simulink model "Scratch3"  (Simulink 8.5)
settings: Solver=ode4  StartTime=0.0  StopTime=20  FixedStep=0.005  RelTol=1e-3
libraries: dspinverses x1, roblocks x1
(part 2 of 3)

== matlab function Christoffle Matrix (C) ==
  data: q1d input double; q2d input double; q3d input double; q4d input double; q1 input double; C_Num output double; q2 input double; q3 input double; q4 input double; q1dd input double; q2dd input double; q3dd input double; q4dd input double; Cdot_Num output double
function [C_Num,Cdot_Num] = fcn(q1d, q2d, q3d, q4d, q1, q2, q3, q4, q1dd, q2dd, q3dd, q4dd)
%#codegen
% coder.extrinsic('evalin');
% coder.extrinsic('subs'); 
% coder.extrinsic('eval'); 
% 
% StatesSym1 = evalin('base','states1');
% StatesSym2 = evalin('base','states2');
% 
% Csym = evalin('base','C');
% Cdotsym = evalin('base','Cdot');
% 
% 
% States_Num1 = [q1t;q2t;q3t;q4t;q1dt;q2dt;q3dt;q4dt];
% States_Num2 = [q1t;q2t;q3t;q4t;q1dt;q2dt;q3dt;q4dt;q1ddt;q2ddt;q3ddt;q4ddt];
% 
% C_Num = zeros(4,1);
% Cdot_Num = zeros(4,1);
% C_Num = eval(subs(Csym,StatesSym1,States_Num1));
% Cdot_Num = eval(subs(Cdotsym,StatesSym2,States_Num2));

m2 = 7;
m3 = 7;
m4 = 5;
l1 = 1;
l2 = 0.7;
l3 = 0.7; 
l4 = 0.5;
d2 = l2/2;
d3 = l3/2; 
d4 = l4/2;


C_Num = [- q4d*(q1d*(d4*l2*m4*sin(q3 + q4) + d4*l3*m4*sin(q4) + d4*l1*m4*sin(q2 + q3 + q4)) + q2d*(d4*l2*m4*sin(q3 + q4) + d4*l3*m4*sin(q4) + d4*l1*m4*sin(q2 + q3 + q4)) + q3d*(d4*l2*m4*sin(q3 + q4) + d4*l3*m4*sin(q4) + d4*l1*m4*sin(q2 + q3 + q4)) + q4d*(d4*l2*m4*sin(q3 + q4) + d4*l3*m4*sin(q4) + d4*l1*m4*sin(q2 + q3 + q4))) - q2d*(q2d*(d3*l1*m3*sin(q2 + q3) - (l1^2*m2*sin(2*q1))/2 - (d2^2*m2*sin(2*q1 + 2*q2))/2 + l1*l3*m4*sin(q2 + q3) + (d2*l1*m2*sin(q2))/2 + l1*l2*m3*sin(q2) + l1*l2*m4*sin(q2) - (d2*l1*m2*sin(2*q1 + q2))/2 + d4*l1*m4*sin(q2 + q3 + q4)) + q4d*(d4*l2*m4*sin(q3 + q4) + d4*l3*m4*sin(q4) + d4*l1*m4*sin(q2 + q3 + q4)) + q1d*(d3*l1*m3*sin(q2 + q3) - (d2^2*m2*sin(2*q1 + 2*q2))/2 + l1*l3*m4*sin(q2 + q3) + (d2*l1*m2*sin(q2))/2 + l1*l2*m3*sin(q2) + l1*l2*m4*sin(q2) - (d2*l1*m2*sin(2*q1 + q2))/2 + d4*l1*m4*sin(q2 + q3 + q4)) + q3d*(d3*l1*m3*sin(q2 + q3) + d4*l2*m4*sin(q3 + q4) + l1*l3*m4*sin(q2 + q3) + d3*l2*m3*sin(q3) + l2*l3*m4*sin(q3) + d4*l1*m4*sin(q2 + q3 + q4))) - q1d*(q4d*(d4*l2*m4*sin(q3 + q4) + d4*l3*m4*sin(q4) + d4*l1*m4*sin(q2 + q3 + q4)) - q1d*((m2*sin(2*q1 + 2*q2)*d2^2)/2 + m2*sin(2*q1 + q2)*d2*l1 + (m2*sin(2*q1)*l1^2)/2) + q2d*(d3*l1*m3*sin(q2 + q3) - (d2^2*m2*sin(2*q1 + 2*q2))/2 + l1*l3*m4*sin(q2 + q3) + (d2*l1*m2*sin(q2))/2 + l1*l2*m3*sin(q2) + l1*l2*m4*sin(q2) - (d2*l1*m2*sin(2*q1 + q2))/2 + d4*l1*m4*sin(q2 + q3 + q4)) + q3d*(d3*l1*m3*sin(q2 + q3) + d4*l2*m4*sin(q3 + q4) + l1*l3*m4*sin(q2 + q3) + d3*l2*m3*sin(q3) + l2*l3*m4*sin(q3) + d4*l1*m4*sin(q2 + q3 + q4))) - q3d*(q4d*(d4*l2*m4*sin(q3 + q4) + d4*l3*m4*sin(q4) + d4*l1*m4*sin(q2 + q3 + q4)) + q1d*(d3*l1*m3*sin(q2 + q3) + d4*l2*m4*sin(q3 + q4) + l1*l3*m4*sin(q2 + q3) + d3*l2*m3*sin(q3) + l2*l3*m4*sin(q3) + d4*l1*m4*sin(q2 + q3 + q4)) + q2d*(d3*l1*m3*sin(q2 + q3) + d4*l2*m4*sin(q3 + q4) + l1*l3*m4*sin(q2 + q3) + d3*l2*m3*sin(q3) + l2*l3*m4*sin(q3) + d4*l1*m4*sin(q2 + q3 + q4)) + q3d*(d3*l1*m3*sin(q2 + q3) + d4*l2*m4*sin(q3 + q4) + l1*l3*m4*sin(q2 + q3) + d3*l2*m3*sin(q3) + l2*l3*m4*sin(q3) + d4*l1*m4*sin(q2 + q3 + q4)))
                                                                                                                                                                                                                                                                                                                                                                                                                                                                                                                                                                                                                                                                                                                                                                                                                                                                                                                                                                                         - q4d*(q1d*(d4*l2*m4*sin(q3 + q4) + d4*l3*m4*sin(q4)) + q2d*(d4*l2*m4*sin(q3 + q4) + d4*l3*m4*sin(q4)) + q3d*(d4*l2*m4*sin(q3 + q4) + d4*l3*m4*sin(q4)) + q4d*(d4*l2*m4*sin(q3 + q4) + d4*l3*m4*sin(q4))) - q2d*(q4d*(d4*l2*m4*sin(q3 + q4) + d4*l3*m4*sin(q4)) - q1d*((m2*sin(2*q1 + 2*q2)*d2^2)/2 - (l1^2*m2*sin(2*q1))/2) + q3d*(d4*l2*m4*sin(q3 + q4) + d3*l2*m3*sin(q3) + l2*l3*m4*sin(q3)) - (d2^2*m2*q2d*sin(2*q1 + 2*q2))/2) - q1d*(q4d*(d4*l2*m4*sin(q3 + q4) + d4*l3*m4*sin(q4)) - q2d*((m2*sin(2*q1 + 2*q2)*d2^2)/2 - (l1^2*m2*sin(2*q1))/2) + q3d*(d4*l2*m4*sin(q3 + q4) + d3*l2*m3*sin(q3) + l2*l3*m4*sin(q3)) - q1d*((d2^2*m2*sin(2*q1 + 2*q2))/2 + d3*l1*m3*sin(q2 + q3) + l1*l3*m4*sin(q2 + q3) + (d2*l1*m2*sin(q2))/2 + l1*l2*m3*sin(q2) + l1*l2*m4*sin(q2) + (d2*l1*m2*sin(2*q1 + q2))/2 + d4*l1*m4*sin(q2 + q3 + q4))) - q3d*(q4d*(d4*l2*m4*sin(q3 + q4) + d4*l3*m4*sin(q4)) + q1d*(d4*l2*m4*sin(q3 + q4) + d3*l2*m3*sin(q3) + l2*l3*m4*sin(q3)) + q2d*(d4*l2*m4*sin(q3 + q4) + d3*l2*m3*sin(q3) + l2*l3*m4*sin(q3)) + q3d*(d4*l2*m4*sin(q3 + q4) + d3*l2*m3*sin(q3) + l2*l3*m4*sin(q3)))
                                                                                                                                                                                                                                                                                                                                                                                                                                                                                                                                                                                                                                                                                                                                                                                                                                                                                                                                                                                                                                                                                                                                                                                                                                                                                                                                                                                                                                                                                                                                                    q2d*(q1d*(d4*l2*m4*sin(q3 + q4) + d3*l2*m3*sin(q3) + l2*l3*m4*sin(q3)) + q2d*(d4*l2*m4*sin(q3 + q4) + d3*l2*m3*sin(q3) + l2*l3*m4*sin(q3)) - d4*l3*m4*q4d*sin(q4)) + q1d*(q2d*(d4*l2*m4*sin(q3 + q4) + d3*l2*m3*sin(q3) + l2*l3*m4*sin(q3)) + q1d*(d3*l1*m3*sin(q2 + q3) + d4*l2*m4*sin(q3 + q4) + l1*l3*m4*sin(q2 + q3) + d3*l2*m3*sin(q3) + l2*l3*m4*sin(q3) + d4*l1*m4*sin(q2 + q3 + q4)) - d4*l3*m4*q4d*sin(q4)) - q4d*(d4*l3*m4*q1d*sin(q4) + d4*l3*m4*q2d*sin(q4) + d4*l3*m4*q3d*sin(q4) + d4*l3*m4*q4d*sin(q4)) - d4*l3*m4*q3d*q4d*sin(q4)
                                                                                                                                                                                                                                                                                                                                                                                                                                                                                                                                                                                                                                                                                                                                                                                                                                                                                                                                                                                                                                                                                                                                                                                                                                                                                                                                                                                                                                                                                                                                                    q2d*(q1d*(d4*l2*m4*sin(q3 + q4) + d3*l2*m3*sin(q3) + l2*l3*m4*sin(q3)) + q2d*(d4*l2*m4*sin(q3 + q4) + d3*l2*m3*sin(q3) + l2*l3*m4*sin(q3)) - d4*l3*m4*q4d*sin(q4)) + q1d*(q2d*(d4*l2*m4*sin(q3 + q4) + d3*l2*m3*sin(q3) + l2*l3*m4*sin(q3)) + q1d*(d3*l1*m3*sin(q2 + q3) + d4*l2*m4*sin(q3 + q4) + l1*l3*m4*sin(q2 + q3) + d3*l2*m3*sin(q3) + l2*l3*m4*sin(q3) + d4*l1*m4*sin(q2 + q3 + q4)) - d4*l3*m4*q4d*sin(q4)) - q4d*(d4*l3*m4*q1d*sin(q4) + d4*l3*m4*q2d*sin(q4) + d4*l3*m4*q3d*sin(q4) + d4*l3*m4*q4d*sin(q4)) - d4*l3*m4*q3d*q4d*sin(q4)];

Cdot_Num = [q1d*(q2d*(q2d*(m2*cos(2*q1 + 2*q2)*d2^2 + m2*cos(2*q1 + q2)*d2*l1 + m2*cos(2*q1)*l1^2) + q1d*(m2*cos(2*q1 + 2*q2)*d2^2 + l1*m2*cos(2*q1 + q2)*d2)) + q1d*(q1d*(m2*cos(2*q1 + 2*q2)*d2^2 + 2*m2*cos(2*q1 + q2)*d2*l1 + m2*cos(2*q1)*l1^2) + q2d*(m2*cos(2*q1 + 2*q2)*d2^2 + l1*m2*cos(2*q1 + q2)*d2))) - q3d*(q3d*(q4d*(d4*l2*m4*cos(q3 + q4) + d4*l1*m4*cos(q2 + q3 + q4)) + q1d*(d3*l1*m3*cos(q2 + q3) + d4*l2*m4*cos(q3 + q4) + l1*l3*m4*cos(q2 + q3) + d3*l2*m3*cos(q3) + l2*l3*m4*cos(q3) + d4*l1*m4*cos(q2 + q3 + q4)) + q2d*(d3*l1*m3*cos(q2 + q3) + d4*l2*m4*cos(q3 + q4) + l1*l3*m4*cos(q2 + q3) + d3*l2*m3*cos(q3) + l2*l3*m4*cos(q3) + d4*l1*m4*cos(q2 + q3 + q4)) + q3d*(d3*l1*m3*cos(q2 + q3) + d4*l2*m4*cos(q3 + q4) + l1*l3*m4*cos(q2 + q3) + d3*l2*m3*cos(q3) + l2*l3*m4*cos(q3) + d4*l1*m4*cos(q2 + q3 + q4))) + q1d*(q4d*(d4*l2*m4*cos(q3 + q4) + d4*l1*m4*cos(q2 + q3 + q4)) + q2d*(d3*l1*m3*cos(q2 + q3) + l1*l3*m4*cos(q2 + q3) + d4*l1*m4*cos(q2 + q3 + q4)) + q3d*(d3*l1*m3*cos(q2 + q3) + d4*l2*m4*cos(q3 + q4) + l1*l3*m4*cos(q2 + q3) + d3*l2*m3*cos(q3) + l2*l3*m4*cos(q3) + d4*l1*m4*cos(q2 + q3 + q4))) + q4d*(q1d*(d4*l2*m4*cos(q3 + q4) + d4*l1*m4*cos(q2 + q3 + q4)) + q2d*(d4*l2*m4*cos(q3 + q4) + d4*l1*m4*cos(q2 + q3 + q4)) + q3d*(d4*l2*m4*cos(q3 + q4) + d4*l1*m4*cos(q2 + q3 + q4)) + q4d*(d4*l2*m4*cos(q3 + q4) + d4*l1*m4*cos(q2 + q3 + q4))) + q2d*(q4d*(d4*l2*m4*cos(q3 + q4) + d4*l1*m4*cos(q2 + q3 + q4)) + q1d*(d3*l1*m3*cos(q2 + q3) + l1*l3*m4*cos(q2 + q3) + d4*l1*m4*cos(q2 + q3 + q4)) + q2d*(d3*l1*m3*cos(q2 + q3) + l1*l3*m4*cos(q2 + q3) + d4*l1*m4*cos(q2 + q3 + q4)) + q3d*(d3*l1*m3*cos(q2 + q3) + d4*l2*m4*cos(q3 + q4) + l1*l3*m4*cos(q2 + q3) + d3*l2*m3*cos(q3) + l2*l3*m4*cos(q3) + d4*l1*m4*cos(q2 + q3 + q4)))) - q4d*(q1d*(q3d*(d4*l2*m4*cos(q3 + q4) + d4*l1*m4*cos(q2 + q3 + q4)) + q4d*(d4*l2*m4*cos(q3 + q4) + d4*l3*m4*cos(q4) + d4*l1*m4*cos(q2 + q3 + q4)) + d4*l1*m4*q2d*cos(q2 + q3 + q4)) + q2d*(q3d*(d4*l2*m4*cos(q3 + q4) + d4*l1*m4*cos(q2 + q3 + q4)) + q4d*(d4*l2*m4*cos(q3 + q4) + d4*l3*m4*cos(q4) + d4*l1*m4*cos(q2 + q3 + q4)) + d4*l1*m4*q1d*cos(q2 + q3 + q4) + d4*l1*m4*q2d*cos(q2 + q3 + q4)) + q3d*(q1d*(d4*l2*m4*cos(q3 + q4) + d4*l1*m4*cos(q2 + q3 + q4)) + q2d*(d4*l2*m4*cos(q3 + q4) + d4*l1*m4*cos(q2 + q3 + q4)) + q3d*(d4*l2*m4*cos(q3 + q4) + d4*l1*m4*cos(q2 + q3 + q4)) + q4d*(d4*l2*m4*cos(q3 + q4) + d4*l3*m4*cos(q4) + d4*l1*m4*cos(q2 + q3 + q4))) + q4d*(q1d*(d4*l2*m4*cos(q3 + q4) + d4*l3*m4*cos(q4) + d4*l1*m4*cos(q2 + q3 + q4)) + q2d*(d4*l2*m4*cos(q3 + q4) + d4*l3*m4*cos(q4) + d4*l1*m4*cos(q2 + q3 + q4)) + q3d*(d4*l2*m4*cos(q3 + q4) + d4*l3*m4*cos(q4) + d4*l1*m4*cos(q2 + q3 + q4)) + q4d*(d4*l2*m4*cos(q3 + q4) + d4*l3*m4*cos(q4) + d4*l1*m4*cos(q2 + q3 + q4)))) - q4dd*(2*q1d*(d4*l2*m4*sin(q3 + q4) + d4*l3*m4*sin(q4) + d4*l1*m4*sin(q2 + q3 + q4)) + 2*q2d*(d4*l2*m4*sin(q3 + q4) + d4*l3*m4*sin(q4) + d4*l1*m4*sin(q2 + q3 + q4)) + 2*q3d*(d4*l2*m4*sin(q3 + q4) + d4*l3*m4*sin(q4) + d4*l1*m4*sin(q2 + q3 + q4)) + 2*q4d*(d4*l2*m4*sin(q3 + q4) + d4*l3*m4*sin(q4) + d4*l1*m4*sin(q2 + q3 + q4))) - q2dd*(2*q2d*(d3*l1*m3*sin(q2 + q3) - (l1^2*m2*sin(2*q1))/2 - (d2^2*m2*sin(2*q1 + 2*q2))/2 + l1*l3*m4*sin(q2 + q3) + (d2*l1*m2*sin(q2))/2 + l1*l2*m3*sin(q2) + l1*l2*m4*sin(q2) - (d2*l1*m2*sin(2*q1 + q2))/2 + d4*l1*m4*sin(q2 + q3 + q4)) + 2*q4d*(d4*l2*m4*sin(q3 + q4) + d4*l3*m4*sin(q4) + d4*l1*m4*sin(q2 + q3 + q4)) + 2*q1d*(d3*l1*m3*sin(q2 + q3) - (d2^2*m2*sin(2*q1 + 2*q2))/2 + l1*l3*m4*sin(q2 + q3) + (d2*l1*m2*sin(q2))/2 + l1*l2*m3*sin(q2) + l1*l2*m4*sin(q2) - (d2*l1*m2*sin(2*q1 + q2))/2 + d4*l1*m4*sin(q2 + q3 + q4)) + 2*q3d*(d3*l1*m3*sin(q2 + q3) + d4*l2*m4*sin(q3 + q4) + l1*l3*m4*sin(q2 + q3) + d3*l2*m3*sin(q3) + l2*l3*m4*sin(q3) + d4*l1*m4*sin(q2 + q3 + q4))) - q1dd*(2*q4d*(d4*l2*m4*sin(q3 + q4) + d4*l3*m4*sin(q4) + d4*l1*m4*sin(q2 + q3 + q4)) - 2*q1d*((m2*sin(2*q1 + 2*q2)*d2^2)/2 + m2*sin(2*q1 + q2)*d2*l1 + (m2*sin(2*q1)*l1^2)/2) + 2*q2d*(d3*l1*m3*sin(q2 + q3) - (d2^2*m2*sin(2*q1 + 2*q2))/2 + l1*l3*m4*sin(q2 + q3) + (d2*l1*m2*sin(q2))/2 + l1*l2*m3*sin(q2) + l1*l2*m4*sin(q2) - (d2*l1*m2*sin(2*q1 + q2))/2 + d4*l1*m4*sin(q2 + q3 + q4)) + 2*q3d*(d3*l1*m3*sin(q2 + q3) + d4*l2*m4*sin(q3 + q4) + l1*l3*m4*sin(q2 + q3) + d3*l2*m3*sin(q3) + l2*l3*m4*sin(q3) + d4*l1*m4*sin(q2 + q3 + q4))) - q3dd*(2*q4d*(d4*l2*m4*sin(q3 + q4) + d4*l3*m4*sin(q4) + d4*l1*m4*sin(q2 + q3 + q4)) + 2*q1d*(d3*l1*m3*sin(q2 + q3) + d4*l2*m4*sin(q3 + q4) + l1*l3*m4*sin(q2 + q3) + d3*l2*m3*sin(q3) + l2*l3*m4*sin(q3) + d4*l1*m4*sin(q2 + q3 + q4)) + 2*q2d*(d3*l1*m3*sin(q2 + q3) + d4*l2*m4*sin(q3 + q4) + l1*l3*m4*sin(q2 + q3) + d3*l2*m3*sin(q3) + l2*l3*m4*sin(q3) + d4*l1*m4*sin(q2 + q3 + q4)) + 2*q3d*(d3*l1*m3*sin(q2 + q3) + d4*l2*m4*sin(q3 + q4) + l1*l3*m4*sin(q2 + q3) + d3*l2*m3*sin(q3) + l2*l3*m4*sin(q3) + d4*l1*m4*sin(q2 + q3 + q4))) - q2d*(q2d*(q1d*(d3*l1*m3*cos(q2 + q3) - d2^2*m2*cos(2*q1 + 2*q2) + l1*l3*m4*cos(q2 + q3) + (d2*l1*m2*cos(q2))/2 + l1*l2*m3*cos(q2) + l1*l2*m4*cos(q2) - (d2*l1*m2*cos(2*q1 + q2))/2 + d4*l1*m4*cos(q2 + q3 + q4)) + q2d*(d3*l1*m3*cos(q2 + q3) - d2^2*m2*cos(2*q1 + 2*q2) + l1*l3*m4*cos(q2 + q3) + (d2*l1*m2*cos(q2))/2 + l1*l2*m3*cos(q2) + l1*l2*m4*cos(q2) - (d2*l1*m2*cos(2*q1 + q2))/2 + d4*l1*m4*cos(q2 + q3 + q4)) + q3d*(d3*l1*m3*cos(q2 + q3) + l1*l3*m4*cos(q2 + q3) + d4*l1*m4*cos(q2 + q3 + q4)) + d4*l1*m4*q4d*cos(q2 + q3 + q4)) + q3d*(q1d*(d3*l1*m3*cos(q2 + q3) + l1*l3*m4*cos(q2 + q3) + d4*l1*m4*cos(q2 + q3 + q4)) + q2d*(d3*l1*m3*cos(q2 + q3) + l1*l3*m4*cos(q2 + q3) + d4*l1*m4*cos(q2 + q3 + q4)) + q3d*(d3*l1*m3*cos(q2 + q3) + l1*l3*m4*cos(q2 + q3) + d4*l1*m4*cos(q2 + q3 + q4)) + d4*l1*m4*q4d*cos(q2 + q3 + q4)) + q4d*(d4*l1*m4*q1d*cos(q2 + q3 + q4) + d4*l1*m4*q2d*cos(q2 + q3 + q4) + d4*l1*m4*q3d*cos(q2 + q3 + q4) + d4*l1*m4*q4d*cos(q2 + q3 + q4)) + q1d*(q2d*(d3*l1*m3*cos(q2 + q3) - d2^2*m2*cos(2*q1 + 2*q2) + l1*l3*m4*cos(q2 + q3) + (d2*l1*m2*cos(q2))/2 + l1*l2*m3*cos(q2) + l1*l2*m4*cos(q2) - (d2*l1*m2*cos(2*q1 + q2))/2 + d4*l1*m4*cos(q2 + q3 + q4)) + q3d*(d3*l1*m3*cos(q2 + q3) + l1*l3*m4*cos(q2 + q3) + d4*l1*m4*cos(q2 + q3 + q4)) - q1d*(m2*cos(2*q1 + 2*q2)*d2^2 + l1*m2*cos(2*q1 + q2)*d2) + d4*l1*m4*q4d*cos(q2 + q3 + q4)))
                                                                                                                                                                                                                                                                                                                                                                                                                                                                                                                                                                                                                                                                                                                                                                                                                                                                                                                                                                                                                                                                                                                                                                                                                                                                                                                                                                                                                                                                                                                                                                                                                                                                                                                                                                                                                                                                                                                                                                                                                                                                                                                                                                                                                                                                                                                                                                                                                                                                                                                                                                                                                                                                                                                                                                                                                                                                                                                                                                                                                                                                                                                                                                                                                                                                                                                                                                                           q2d*(q1d*(q1d*(d2^2*m2*cos(2*q1 + 2*q2) + d3*l1*m3*cos(q2 + q3) + l1*l3*m4*cos(q2 + q3) + (d2*l1*m2*cos(q2))/2 + l1*l2*m3*cos(q2) + l1*l2*m4*cos(q2) + (d2*l1*m2*cos(2*q1 + q2))/2 + d4*l1*m4*cos(q2 + q3 + q4)) + d2^2*m2*q2d*cos(2*q1 + 2*q2)) + q2d*(d2^2*m2*q1d*cos(2*q1 + 2*q2) + d2^2*m2*q2d*cos(2*q1 + 2*q2))) - q3d*(q2d*(q3d*(d4*l2*m4*cos(q3 + q4) + d3*l2*m3*cos(q3) + l2*l3*m4*cos(q3)) + d4*l2*m4*q4d*cos(q3 + q4)) + q1d*(q3d*(d4*l2*m4*cos(q3 + q4) + d3*l2*m3*cos(q3) + l2*l3*m4*cos(q3)) - q1d*(d3*l1*m3*cos(q2 + q3) + l1*l3*m4*cos(q2 + q3) + d4*l1*m4*cos(q2 + q3 + q4)) + d4*l2*m4*q4d*cos(q3 + q4)) + q3d*(q1d*(d4*l2*m4*cos(q3 + q4) + d3*l2*m3*cos(q3) + l2*l3*m4*cos(q3)) + q2d*(d4*l2*m4*cos(q3 + q4) + d3*l2*m3*cos(q3) + l2*l3*m4*cos(q3)) + q3d*(d4*l2*m4*cos(q3 + q4) + d3*l2*m3*cos(q3) + l2*l3*m4*cos(q3)) + d4*l2*m4*q4d*cos(q3 + q4)) + q4d*(d4*l2*m4*q1d*cos(q3 + q4) + d4*l2*m4*q2d*cos(q3 + q4) + d4*l2*m4*q3d*cos(q3 + q4) + d4*l2*m4*q4d*cos(q3 + q4))) - q4dd*(2*q1d*(d4*l2*m4*sin(q3 + q4) + d4*l3*m4*sin(q4)) + 2*q2d*(d4*l2*m4*sin(q3 + q4) + d4*l3*m4*sin(q4)) + 2*q3d*(d4*l2*m4*sin(q3 + q4) + d4*l3*m4*sin(q4)) + 2*q4d*(d4*l2*m4*sin(q3 + q4) + d4*l3*m4*sin(q4))) - q2dd*(2*q4d*(d4*l2*m4*sin(q3 + q4) + d4*l3*m4*sin(q4)) - 2*q1d*((m2*sin(2*q1 + 2*q2)*d2^2)/2 - (l1^2*m2*sin(2*q1))/2) + 2*q3d*(d4*l2*m4*sin(q3 + q4) + d3*l2*m3*sin(q3) + l2*l3*m4*sin(q3)) - d2^2*m2*q2d*sin(2*q1 + 2*q2)) - q1d*(q2d*(q1d*(m2*cos(2*q1)*l1^2 - m2*cos(2*q1 + 2*q2)*d2^2) - d2^2*m2*q2d*cos(2*q1 + 2*q2)) - q1d*(q1d*(m2*cos(2*q1 + 2*q2)*d2^2 + l1*m2*cos(2*q1 + q2)*d2) - q2d*(m2*cos(2*q1)*l1^2 - m2*cos(2*q1 + 2*q2)*d2^2))) - q1dd*(2*q4d*(d4*l2*m4*sin(q3 + q4) + d4*l3*m4*sin(q4)) - 2*q2d*((m2*sin(2*q1 + 2*q2)*d2^2)/2 - (l1^2*m2*sin(2*q1))/2) + 2*q3d*(d4*l2*m4*sin(q3 + q4) + d3*l2*m3*sin(q3) + l2*l3*m4*sin(q3)) - 2*q1d*((d2^2*m2*sin(2*q1 + 2*q2))/2 + d3*l1*m3*sin(q2 + q3) + l1*l3*m4*sin(q2 + q3) + (d2*l1*m2*sin(q2))/2 + l1*l2*m3*sin(q2) + l1*l2*m4*sin(q2) + (d2*l1*m2*sin(2*q1 + q2))/2 + d4*l1*m4*sin(q2 + q3 + q4))) - q4d*(q3d*(q4d*(d4*l2*m4*cos(q3 + q4) + d4*l3*m4*cos(q4)) + d4*l2*m4*q1d*cos(q3 + q4) + d4*l2*m4*q2d*cos(q3 + q4) + d4*l2*m4*q3d*cos(q3 + q4)) + q4d*(q1d*(d4*l2*m4*cos(q3 + q4) + d4*l3*m4*cos(q4)) + q2d*(d4*l2*m4*cos(q3 + q4) + d4*l3*m4*cos(q4)) + q3d*(d4*l2*m4*cos(q3 + q4) + d4*l3*m4*cos(q4)) + q4d*(d4*l2*m4*cos(q3 + q4) + d4*l3*m4*cos(q4))) + q2d*(q4d*(d4*l2*m4*cos(q3 + q4) + d4*l3*m4*cos(q4)) + d4*l2*m4*q3d*cos(q3 + q4)) + q1d*(q4d*(d4*l2*m4*cos(q3 + q4) + d4*l3*m4*cos(q4)) - d4*l1*m4*q1d*cos(q2 + q3 + q4) + d4*l2*m4*q3d*cos(q3 + q4))) - q3dd*(2*q4d*(d4*l2*m4*sin(q3 + q4) + d4*l3*m4*sin(q4)) + 2*q1d*(d4*l2*m4*sin(q3 + q4) + d3*l2*m3*sin(q3) + l2*l3*m4*sin(q3)) + 2*q2d*(d4*l2*m4*sin(q3 + q4) + d3*l2*m3*sin(q3) + l2*l3*m4*sin(q3)) + 2*q3d*(d4*l2*m4*sin(q3 + q4) + d3*l2*m3*sin(q3) + l2*l3*m4*sin(q3)))
                                                                                                                                                                                                                                                                                                                                                                                                                                                                                                                                                                                                                                                                                                                                                                                                                                                                                                                                                                                                                                                                                                                                                                                                                                                                                                                                                                                                                                                                                                                                                                                                                                                                                                                                                                                                                                                                                                                                                                                                                                                                                                                                                                                                                                                                                                                                                                                                                                                                                                                                                                                                                                                                                                                                                                                                                                                                                                                                                                                                                                                                                                                                                                                                                                                                                                                                                                                                                                                                                                                                                                                                                                                                                                                                                                                                                                                                                                                                                                                                                                                                                                                                                                                                                                                                                                                                                                                                                                                                                                                                                                                                                                                                                                                                                                                                                                                                                                                             q2dd*(2*q1d*(d4*l2*m4*sin(q3 + q4) + d3*l2*m3*sin(q3) + l2*l3*m4*sin(q3)) + 2*q2d*(d4*l2*m4*sin(q3 + q4) + d3*l2*m3*sin(q3) + l2*l3*m4*sin(q3)) - 2*d4*l3*m4*q4d*sin(q4)) + q3d*(q1d*(q2d*(d4*l2*m4*cos(q3 + q4) + d3*l2*m3*cos(q3) + l2*l3*m4*cos(q3)) + q1d*(d3*l1*m3*cos(q2 + q3) + d4*l2*m4*cos(q3 + q4) + l1*l3*m4*cos(q2 + q3) + d3*l2*m3*cos(q3) + l2*l3*m4*cos(q3) + d4*l1*m4*cos(q2 + q3 + q4))) + q2d*(q1d*(d4*l2*m4*cos(q3 + q4) + d3*l2*m3*cos(q3) + l2*l3*m4*cos(q3)) + q2d*(d4*l2*m4*cos(q3 + q4) + d3*l2*m3*cos(q3) + l2*l3*m4*cos(q3)))) + q4d*(q2d*(d4*l2*m4*q1d*cos(q3 + q4) + d4*l2*m4*q2d*cos(q3 + q4) - d4*l3*m4*q4d*cos(q4)) - q4d*(d4*l3*m4*q1d*cos(q4) + d4*l3*m4*q2d*cos(q4) + d4*l3*m4*q3d*cos(q4) + d4*l3*m4*q4d*cos(q4)) + q1d*(q1d*(d4*l2*m4*cos(q3 + q4) + d4*l1*m4*cos(q2 + q3 + q4)) + d4*l2*m4*q2d*cos(q3 + q4) - d4*l3*m4*q4d*cos(q4)) - d4*l3*m4*q3d*q4d*cos(q4)) + q1dd*(2*q2d*(d4*l2*m4*sin(q3 + q4) + d3*l2*m3*sin(q3) + l2*l3*m4*sin(q3)) + 2*q1d*(d3*l1*m3*sin(q2 + q3) + d4*l2*m4*sin(q3 + q4) + l1*l3*m4*sin(q2 + q3) + d3*l2*m3*sin(q3) + l2*l3*m4*sin(q3) + d4*l1*m4*sin(q2 + q3 + q4)) - 2*d4*l3*m4*q4d*sin(q4)) - q4dd*(2*d4*l3*m4*q1d*sin(q4) + 2*d4*l3*m4*q2d*sin(q4) + 2*d4*l3*m4*q3d*sin(q4) + 2*d4*l3*m4*q4d*sin(q4)) + q1d^2*q2d*(d3*l1*m3*cos(q2 + q3) + l1*l3*m4*cos(q2 + q3) + d4*l1*m4*cos(q2 + q3 + q4)) - 2*d4*l3*m4*q4d*q3dd*sin(q4)
                                                                                                                                                                                                                                                                                                                                                                                                                                                                                                                                                                                                                                                                                                                                                                                                                                                                                                                                                                                                                                                                                                                                                                                                                                                                                                                                                                                                                                                                                                                                                                                                                                                                                                                                                                                                                                                                                                                                                                                                                                                                                                                                                                                                                                                                                                                                                                                                                                                                                                                                                                                                                                                                                                                                                                                                                                                                                                                                                                                                                                                                                                                                                                                                                                                                                                                                                                                                                                                                                                                                                                                                                                                                                                                                                                                                                                                                                                                                                                                                                                                                                                                                                                                                                                                                                                                                                                                                                                                                                                                                                                                                                                                                                                                                                                                                                                                                                                                             q2dd*(2*q1d*(d4*l2*m4*sin(q3 + q4) + d3*l2*m3*sin(q3) + l2*l3*m4*sin(q3)) + 2*q2d*(d4*l2*m4*sin(q3 + q4) + d3*l2*m3*sin(q3) + l2*l3*m4*sin(q3)) - 2*d4*l3*m4*q4d*sin(q4)) + q3d*(q1d*(q2d*(d4*l2*m4*cos(q3 + q4) + d3*l2*m3*cos(q3) + l2*l3*m4*cos(q3)) + q1d*(d3*l1*m3*cos(q2 + q3) + d4*l2*m4*cos(q3 + q4) + l1*l3*m4*cos(q2 + q3) + d3*l2*m3*cos(q3) + l2*l3*m4*cos(q3) + d4*l1*m4*cos(q2 + q3 + q4))) + q2d*(q1d*(d4*l2*m4*cos(q3 + q4) + d3*l2*m3*cos(q3) + l2*l3*m4*cos(q3)) + q2d*(d4*l2*m4*cos(q3 + q4) + d3*l2*m3*cos(q3) + l2*l3*m4*cos(q3)))) + q4d*(q2d*(d4*l2*m4*q1d*cos(q3 + q4) + d4*l2*m4*q2d*cos(q3 + q4) - d4*l3*m4*q4d*cos(q4)) - q4d*(d4*l3*m4*q1d*cos(q4) + d4*l3*m4*q2d*cos(q4) + d4*l3*m4*q3d*cos(q4) + d4*l3*m4*q4d*cos(q4)) + q1d*(q1d*(d4*l2*m4*cos(q3 + q4) + d4*l1*m4*cos(q2 + q3 + q4)) + d4*l2*m4*q2d*cos(q3 + q4) - d4*l3*m4*q4d*cos(q4)) - d4*l3*m4*q3d*q4d*cos(q4)) + q1dd*(2*q2d*(d4*l2*m4*sin(q3 + q4) + d3*l2*m3*sin(q3) + l2*l3*m4*sin(q3)) + 2*q1d*(d3*l1*m3*sin(q2 + q3) + d4*l2*m4*sin(q3 + q4) + l1*l3*m4*sin(q2 + q3) + d3*l2*m3*sin(q3) + l2*l3*m4*sin(q3) + d4*l1*m4*sin(q2 + q3 + q4)) - 2*d4*l3*m4*q4d*sin(q4)) - q4dd*(2*d4*l3*m4*q1d*sin(q4) + 2*d4*l3*m4*q2d*sin(q4) + 2*d4*l3*m4*q3d*sin(q4) + 2*d4*l3*m4*q4d*sin(q4)) + q1d^2*q2d*(d3*l1*m3*cos(q2 + q3) + l1*l3*m4*cos(q2 + q3) + d4*l1*m4*cos(q2 + q3 + q4)) - 2*d4*l3*m4*q4d*q3dd*sin(q4)];
